simulink model "q6"  (R2021b)
settings: Solver=VariableStepAuto  StartTime=0.0  StopTime=10.0  RelTol=1e-3
libraries: eeGeneralControl x1
settings Model: Creator=Zahra Iranpour  LastModifiedBy=Zahra Iranpour

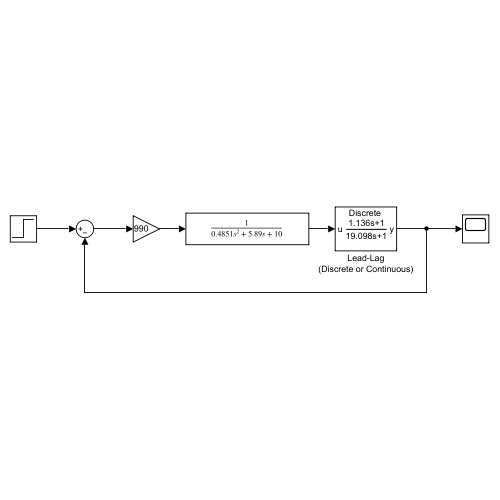
[thumbnail: Simulink's stored preview of the top-level diagram]
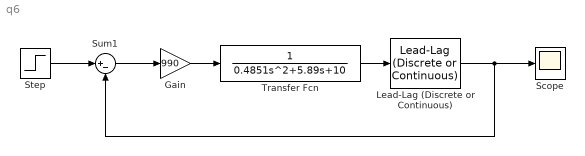
== system q6 ==
  Gain : Gain  Gain=990
  Lead-Lag (Discrete or Continuous) : eeGeneralControl/Lead-Lag (Discrete or Continuous)  T1=1.136  T2=19.098  B=inf  A=-inf  init_option=Inherited from block input  x0=0  Ts=-1
      settings: SourceProductBaseCode=PS
  Scope : Scope
  Step : Step  SampleTime=0
  Sum1 : Sum  Inputs=|+-
  Transfer Fcn : TransferFcn  Denominator=[0.4851 5.89 10]
  wires:
  Lead-Lag (Discrete or Continuous)/1 -> Sum1/2, Scope/1
  Transfer Fcn/1 -> Lead-Lag (Discrete or Continuous)/1
  Gain/1 -> Transfer Fcn/1
  Sum1/1 -> Gain/1
  Step/1 -> Sum1/1
